simulink model "ce"  (R2016b)
settings: Solver=ode4  StartTime=0.0  StopTime=inf  FixedStep=0.001  RelTol=1e-3  EnableMultiTasking=on
undefined symbols (not defined in the file or in its folder): mdaadlink6208
libraries: dsparch4 x10
settings Model: SimulationMode=external  Creator=SHA  LastModifiedBy=Administrator
settings SolverCC: EnableConcurrentExecution=on
settings DataIOCC: SaveFormat=StructureWithTime
settings OptimizationCC: BlockReduction=off  OptimizeBlockIOStorage=off  BufferReuse=off  GlobalBufferReuse=off  ExpressionFolding=off  LocalBlockOutputs=off
settings HardwareCC: ProdBitPerPointer=32  ProdBitPerSizeT=32  ProdBitPerPtrDiffT=32  ProdLargestAtomicFloat=None  ProdWordSize=32  ProdLongLongMode=on  ProdHWDeviceType=Generic->32-bit x86 compatible
settings RTWCC: SystemTargetFile=slrt.tlc  TemplateMakefile=slrt_default_tmf  Description=Simulink Real-Time  RTWCompilerOptimization=on

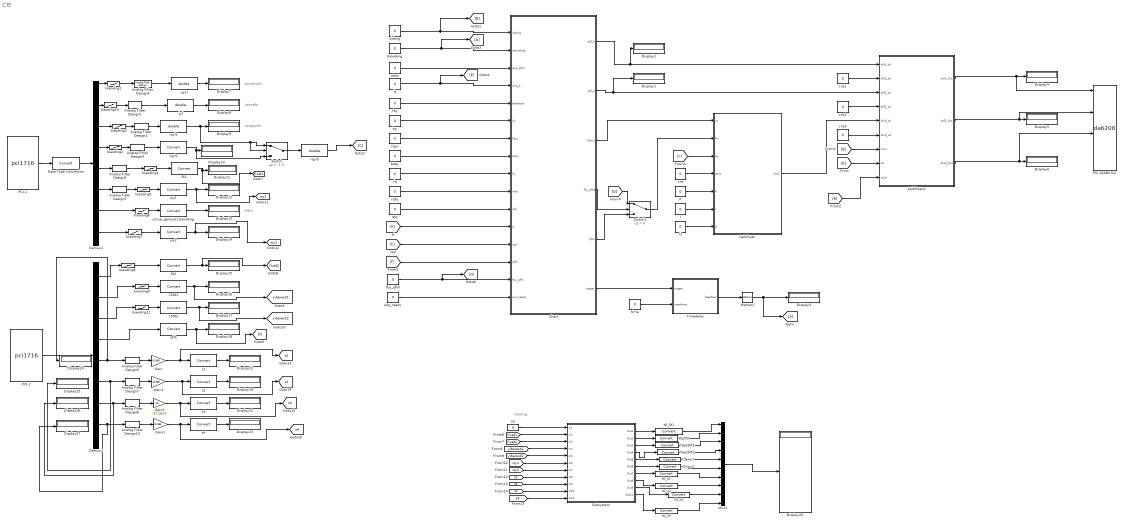
== system ce ==
  note: tiaoling
  note: qiyuanyali
  note: jianyafa
  note: rongqiyali
  note: weiyi
  150t1 : DataTypeConversion
  150t2 : DataTypeConversion
  5t1 : DataTypeConversion
  5t2 : DataTypeConversion
  Analog Filter Design{1..6} (6 alike) : dsparch4/Analog Filter Design  method=Butterworth  filttype=Lowpass  N=8  Wlo=2*pi*25  Whi=80  Rp=2  Rs=40
  Analog Filter Design{7..10} (4 alike) : dsparch4/Analog Filter Design  method=Butterworth  filttype=Lowpass  N=8  Wlo=2*pi*30  Whi=80  Rp=2  Rs=40
  Chart : Stateflow chart  TreatAsAtomicUnit=on
  D : Constant  Value=0
  Data Type Conversion : DataTypeConversion
  Demux1 : Demux  Outputs=16
  Demux2 : Demux  Outputs=16
  Display{1..27} (27 alike) : Display
  Gain : Gain  Gain=42.985
  Gain1 : Gain  Gain=42.985
  Gain2 : Gain  Gain=42.985
  Gain3 : Gain  Gain=-97.0874
  I : Constant  Value=0
  Memory : Memory
  Mux1 : Mux  Inputs=10
  P : Constant  Value=0
  PCI-1 : S-Function  FunctionName=pci1716  Parameters=[SampleTime SampleOffset], SLOT  SFunctionDeploymentMode=off  EnableBusSupport=off  mask(hitad3){Sample=0.001, SLOT=[2 13]}
      mask prompts: Sample "Sample Time:"
      mask help:
      | PCi1716
      | A/D Card
      | Developed by ZhaoJinsong
      | 2012.06.02
      mask init:
      | SampleTime = 0.001; SampleOffset=0;
      mask Help: helpview([docroot '/toolbox/xpc/pt_io_block_reference.html#xpcioref'])
      mask Display:
      | disp('PCI1716  ');
      | 
      | port_label('output',1 , 'OUT');
  PCI-2 : S-Function  FunctionName=pci1716  Parameters=[SampleTime SampleOffset], SLOT  SFunctionDeploymentMode=off  EnableBusSupport=off  mask(hitad3){Sample=0.001, SLOT=[2 12]}
      mask prompts: Sample "Sample Time:"
      mask help:
      | PCi1716
      | A/D Card
      | Developed by ZhaoJinsong
      | 2012.06.02
      mask init:
      | SampleTime = 0.001; SampleOffset=0;
      mask Help: helpview([docroot '/toolbox/xpc/pt_io_block_reference.html#xpcioref'])
      mask Display:
      | disp('PCI1716  ');
      | 
      | port_label('output',1 , 'OUT');
  "PCI-6208A DA " : S-Function  InitFcn=mdaadlink6208( 1 );  FunctionName=da6208  Parameters=channel, range, sampletime, pcislot, reset, initval  SFunctionDeploymentMode=off  EnableBusSupport=off  mask(da6208){channel=[1:8], range=4 to 20 ma, reset=[0], initval=[0], sampletime=0.001, pcislot=-1}
      mask prompts: channel "Channel vector:"; reset "Reset vector:"; initval "Initial value vector:"; sampletime "Sample time:"; pcislot "PCI slot (-1: autosearch):"
      mask help:
      | PCI-6208A
      | Adlink
      | Analog Output
      mask init:
      | [maskdisplay, reset, initval]= mdaadlink6208(2, channel, reset, initval, pcislot);
      | set_param(gcb,'MaskDisplay',maskdisplay);
      mask Help: helpview(fullfile(docroot, 'mapfiles', 'xpc.map'), 'Adlink_6208A_DA')
      mask TypeOptions range: 0 to 20 ma | 5 to 25 ma | 4 to 20 ma
      mask Display: disp('PCI-6208A\nAdlink\nAnalog Output');port_label('input',1,'1');port_label('input',2,'2');port_label('input',3,'3');port_label('input',4,'4');port_label('input',5,'5');port_label('input',6,'6');port_label('input',7,'7');port_label('input',8,'8');
  Subsystem : Subsystem
  Switch : Switch  Criteria=u2 > Threshold  Threshold=-1.5
  Switch1 : Switch  Criteria=u2 > Threshold
  Timedelay : Subsystem
  bdqy : Constant  Value=0
  biaoding{1..3,10} (4 alike) : Lookup  InputValues=[0 5]  Table=[0.01 2]  SaturateOnIntegerOverflow=on
  biaoding11 : Lookup  InputValues=[0 10]  Table=[0 150]  SaturateOnIntegerOverflow=on
  biaoding4 : Lookup  InputValues=[-0.16 10]  Table=[0 5]  SaturateOnIntegerOverflow=on
  biaoding5 : Lookup  InputValues=[-0.063 5]  Table=[0 100]  SaturateOnIntegerOverflow=on
  biaoding6 : Lookup  InputValues=[-0.052 5]  Table=[0 100]  SaturateOnIntegerOverflow=on
  biaoding7 : Lookup  InputValues=[-0.065 5]  Table=[0 100]  SaturateOnIntegerOverflow=on
  biaoding8 : Lookup  InputValues=[-0.002 10]  Table=[0 5]  SaturateOnIntegerOverflow=on
  biaoding9 : Lookup  InputValues=[0 10]  Table=[0 150]  SaturateOnIntegerOverflow=on
  by : Constant  Value=0
  cns{,1..3} (4 alike) : Constant  Value=0
  exp_ready : Constant  Value=0
  fby : Constant  Value=0
  fby_qfkk : Constant  Value=0
  fq : Constant  Value=0
  fqyc : Constant  Value=0
  jt : Constant  Value=0
  jyf : DataTypeConversion  OutDataTypeStr=double
  kaibihuan : Subsystem
  kaibihuan1 : Subsystem
  qffk : DataTypeConversion
  qfq : Constant  Value=0
  qyyl : DataTypeConversion  OutDataTypeStr=double
  rqfq : Constant  Value=0
  rqyl1 : DataTypeConversion  OutDataTypeStr=double
  rqyl2 : DataTypeConversion
  rqyl3 : DataTypeConversion  OutDataTypeStr=double
  s{1..4} (4 alike) : DataTypeConversion
  shoudong : Constant  Value=0
  start : Constant  Value=0
  t0 : Constant  Value=0
  t0_150t1 : DataTypeConversion
  t0_150t2 : DataTypeConversion
  t0_5t1 : DataTypeConversion
  t0_5t2 : DataTypeConversion
  t0_s{1..4} (4 alike) : DataTypeConversion
  t0_wy1 : DataTypeConversion
  t0_wy2 : DataTypeConversion
  time : Constant  Value=0
  wy1 : DataTypeConversion
  wy2 : DataTypeConversion
  yihuai_gensui11biandong : DataTypeConversion
  zidong : Constant  Value=0
  tag scope: fivet1=global, fivet2=global, s1=global, s2=global, s3=global, s4=global, wy1=global, wy2=global, yibaiwut1=global, yibaiwut2=global
  wires:
  start/1 -> Chart/3(exp_start)
  jt/1 -> [E], Chart/4(exp_jt)
  fby/1 -> Chart/5(feibaoya)
  by/1 -> Chart/6(by)
  fqyc/1 -> Chart/7(fqyc)
  Chart/3(kbhxz) -> kaibihuan/1(xz)
  Chart/2(dcf_2) -> kaibihuan1/3(dcf2_zd), Display1/1
  time/1 -> Timedelay/2(needtime)
  fq/1 -> Chart/9(fq)
  Chart/6(trigger) -> Timedelay/1(trigger)
  Timedelay/1(feedbool) -> Memory/1
  Memory/1 -> [A], Display3/1
  cns/1 -> kaibihuan/4(cons)
  P/1 -> kaibihuan/5(P)
  [A] -> Chart/12(sj)
  zidong/1 -> Chart/1(zidong), [B]
  I/1 -> kaibihuan/6(I)
  D/1 -> kaibihuan/7(D)
  [B] -> kaibihuan1/7(kzxz)
  cns1/1 -> kaibihuan1/2(dcf1_sd)
  cns2/1 -> kaibihuan1/4(dcf2_sd)
  cns3/1 -> kaibihuan1/6(dkqf_sd)
  kaibihuan/1(Out1) -> kaibihuan1/5(dkqf_zd)
  Chart/1(dcf_1) -> Display2/1, kaibihuan1/1(dcf1_zd)
  [C] -> Chart/13(rqyl)
  [C] -> kaibihuan/3(qy)
  qfq/1 -> Chart/11(qfq)
  rqfq/1 -> Chart/10(rqfq)
  kaibihuan1/1(dcf1_Out) -> "PCI-6208A DA "/1, Display4/1
  kaibihuan1/2(dcf2_Out) -> "PCI-6208A DA "/3, Display5/1
  kaibihuan1/3(dkqf_Out) -> "PCI-6208A DA "/5, Display6/1
  shoudong/1 -> Chart/2(shoudong), [D]
  Demux1/1 -> biaoding1/1
  Demux1/3 -> biaoding10/1
  Demux1/7 -> biaoding2/1
  PCI-1/1 -> Data Type Conversion/1
  Data Type Conversion/1 -> Demux1/1
  biaoding1/1 -> Analog Filter Design3/1
  biaoding3/1 -> Analog Filter Design2/1
  biaoding5/1 -> wy1/1
  biaoding10/1 -> Analog Filter Design1/1
  qyyl/1 -> Display7/1
  jyf/1 -> Display8/1
  rqyl2/1 -> Switch/3, Display10/1
  5t1/1 -> [fivet1], Display11/1
  wy1/1 -> [wy1], Display12/1
  biaoding6/1 -> yihuai_gensui11biandong/1
  yihuai_gensui11biandong/1 -> Display13/1
  biaoding7/1 -> wy2/1
  wy2/1 -> [wy2], Display14/1
  Demux1/15 -> biaoding7/1
  PCI-2/1 -> Demux2/1
  biaoding9/1 -> 150t1/1
  biaoding11/1 -> 150t2/1
  150t2/1 -> [yibaiwut2], Display17/1
  150t1/1 -> [yibaiwut1], Display16/1
  5t2/1 -> [fivet2], Display15/1
  Demux2/7 -> qffk/1
  qffk/1 -> [F], Display18/1
  [D] -> kaibihuan1/8(sd)
  [E] -> kaibihuan1/9(sd_jt)
  biaoding2/1 -> Analog Filter Design4/1
  Analog Filter Design2/1 -> rqyl1/1
  Analog Filter Design4/1 -> rqyl2/1
  Analog Filter Design1/1 -> jyf/1
  Analog Filter Design3/1 -> qyyl/1
  rqyl1/1 -> Switch/1, Switch/2, Display9/1
  bdqy/1 -> Chart/8(bdqy)
  Switch/1 -> rqyl3/1
  [F] -> Chart/14(qffk)
  fby_qfkk/1 -> [G], Chart/15(fby_qfkk)
  Chart/4(fby_qfsd) -> Switch1/2
  Chart/5(qfkk) -> Switch1/3
  Switch1/1 -> kaibihuan/2(kh)
  [G] -> Switch1/1
  exp_ready/1 -> Chart/16(exp_ready)
  rqyl3/1 -> [C]
  Mux1/1 -> Display20/1
  t0_5t1/1 -> Mux1/1
  t0_5t2/1 -> Mux1/2
  t0_150t1/1 -> Mux1/3
  t0_150t2/1 -> Mux1/4
  t0/1 -> Subsystem/1(In1)
  [fivet1] -> Subsystem/2(In2)
  [fivet2] -> Subsystem/3(In3)
  [yibaiwut1] -> Subsystem/4(In4)
  [yibaiwut2] -> Subsystem/5(In5)
  Subsystem/1(Out1) -> t0_5t1/1
  Subsystem/2(Out2) -> t0_5t2/1
  Subsystem/3(Out3) -> t0_150t1/1
  Subsystem/4(Out4) -> t0_150t2/1
  biaoding4/1 -> 5t1/1
  Demux2/1 -> biaoding8/1
  Demux1/9 -> Analog Filter Design6/1
  Demux1/5 -> biaoding3/1
  s1/1 -> Display22/1
  Gain/1 -> [s1], s1/1
  Demux2/9 -> Display24/1, Analog Filter Design9/1
  Demux2/3 -> biaoding9/1
  Demux2/5 -> biaoding11/1
  [wy1] -> Subsystem/6(In6)
  [wy2] -> Subsystem/7(In7)
  Subsystem/5(Out5) -> t0_wy1/1
  Subsystem/6(Out6) -> t0_wy2/1
  t0_wy1/1 -> Mux1/5
  t0_wy2/1 -> Mux1/6
  Demux1/11 -> Analog Filter Design5/1
  Demux1/13 -> biaoding6/1
  biaoding8/1 -> 5t2/1
  Analog Filter Design5/1 -> biaoding5/1
  Analog Filter Design6/1 -> biaoding4/1
  Gain2/1 -> [s2], s2/1
  Demux2/11 -> Display25/1, Analog Filter Design7/1
  Gain3/1 -> [s3], s3/1
  Gain1/1 -> [s4], s4/1
  Demux2/13 -> Display26/1, Analog Filter Design8/1
  Demux2/15 -> Display27/1, Analog Filter Design10/1
  s4/1 -> Display23/1
  s3/1 -> Display21/1
  s2/1 -> Display19/1
  [s1] -> Subsystem/8(In8)
  [s2] -> Subsystem/9(In9)
  [s3] -> Subsystem/10(In10)
  [s4] -> Subsystem/11(In11)
  t0_s1/1 -> Mux1/7
  t0_s2/1 -> Mux1/8
  t0_s3/1 -> Mux1/9
  t0_s4/1 -> Mux1/10
  Subsystem/7(Out7) -> t0_s1/1
  Subsystem/8(Out8) -> t0_s2/1
  Subsystem/9(Out9) -> t0_s3/1
  Subsystem/10(Out10) -> t0_s4/1
  Analog Filter Design7/1 -> Gain2/1
  Analog Filter Design8/1 -> Gain3/1
  Analog Filter Design9/1 -> Gain/1
  Analog Filter Design10/1 -> Gain1/1

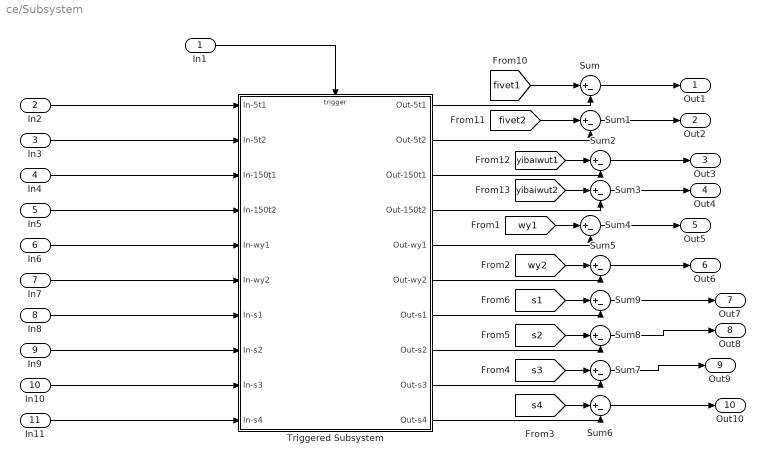
== system ce/Subsystem ==
  In1 : Inport
  In2 : Inport  Port=2
  In3 : Inport  Port=3
  In4 : Inport  Port=4
  In5 : Inport  Port=5
  In6 : Inport  Port=6
  In7 : Inport  Port=7
  In8 : Inport  Port=8
  In9 : Inport  Port=9
  In10 : Inport  Port=10
  In11 : Inport  Port=11
  Sum{,1..9} (10 alike) : Sum  Inputs=|+-
  Triggered Subsystem : Subsystem  TreatAsAtomicUnit=on
  Out1 : Outport
  Out2 : Outport  Port=2
  Out3 : Outport  Port=3
  Out4 : Outport  Port=4
  Out5 : Outport  Port=5
  Out6 : Outport  Port=6
  Out7 : Outport  Port=7
  Out8 : Outport  Port=8
  Out9 : Outport  Port=9
  Out10 : Outport  Port=10
  wires:
  In2/1 -> Triggered Subsystem/1(In-5t1)
  In4/1 -> Triggered Subsystem/3(In-150t1)
  [fivet2] -> Sum1/1
  In3/1 -> Triggered Subsystem/2(In-5t2)
  Triggered Subsystem/3(Out-150t1) -> Sum2/2
  [fivet1] -> Sum/1
  Sum/1 -> Out1/1
  Sum1/1 -> Out2/1
  Sum3/1 -> Out4/1
  Sum2/1 -> Out3/1
  [yibaiwut2] -> Sum3/1
  [yibaiwut1] -> Sum2/1
  Triggered Subsystem/2(Out-5t2) -> Sum1/2
  In5/1 -> Triggered Subsystem/4(In-150t2)
  Triggered Subsystem/1(Out-5t1) -> Sum/2
  In1/1 -> Triggered Subsystem/Trigger
  Triggered Subsystem/4(Out-150t2) -> Sum3/2
  Sum4/1 -> Out5/1
  [wy1] -> Sum4/1
  Triggered Subsystem/5(Out-wy1) -> Sum4/2
  Sum5/1 -> Out6/1
  [wy2] -> Sum5/1
  Triggered Subsystem/6(Out-wy2) -> Sum5/2
  In6/1 -> Triggered Subsystem/5(In-wy1)
  In7/1 -> Triggered Subsystem/6(In-wy2)
  In11/1 -> Triggered Subsystem/10(In-s4)
  In10/1 -> Triggered Subsystem/9(In-s3)
  In9/1 -> Triggered Subsystem/8(In-s2)
  In8/1 -> Triggered Subsystem/7(In-s1)
  Sum6/1 -> Out10/1
  [s4] -> Sum6/1
  Triggered Subsystem/10(Out-s4) -> Sum6/2
  Sum7/1 -> Out9/1
  [s3] -> Sum7/1
  Triggered Subsystem/9(Out-s3) -> Sum7/2
  Sum8/1 -> Out8/1
  [s2] -> Sum8/1
  Triggered Subsystem/8(Out-s2) -> Sum8/2
  Sum9/1 -> Out7/1
  [s1] -> Sum9/1
  Triggered Subsystem/7(Out-s1) -> Sum9/2

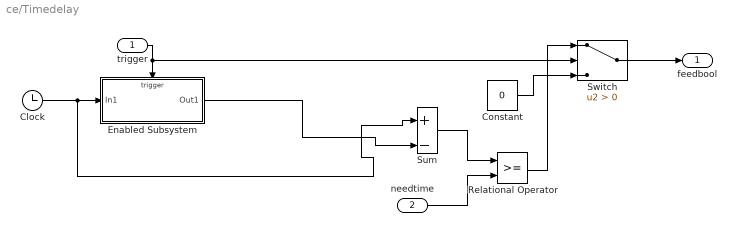
== system ce/Timedelay ==
  trigger : Inport
  needtime : Inport  Port=2
  Clock : Clock
  Constant : Constant  Value=0
  Enabled Subsystem : Subsystem  TreatAsAtomicUnit=on
  Relational Operator : RelationalOperator  OutDataTypeStr=boolean  RndMeth=Simplest
  Sum : Sum  Inputs=|+-
  Switch : Switch  Criteria=u2 > Threshold
  feedbool : Outport
  wires:
  Clock/1 -> Sum/1, Enabled Subsystem/1(In1)
  Enabled Subsystem/1(Out1) -> Sum/2
  Sum/1 -> Relational Operator/1
  needtime/1 -> Relational Operator/2
  trigger/1 -> Switch/2, Enabled Subsystem/Trigger
  Relational Operator/1 -> Switch/1
  Constant/1 -> Switch/3
  Switch/1 -> feedbool/1

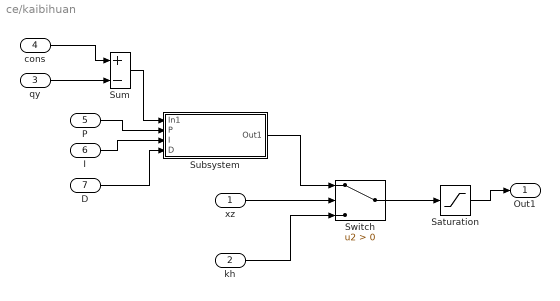
== system ce/kaibihuan ==
  xz : Inport
  kh : Inport  Port=2
  qy : Inport  Port=3
  cons : Inport  Port=4
  P : Inport  Port=5
  I : Inport  Port=6
  D : Inport  Port=7
  Saturation : Saturate  UpperLimit=5  LowerLimit=0
  Subsystem : Subsystem
  Sum : Sum  Inputs=|+-
  Switch : Switch  Criteria=u2 > Threshold
  Out1 : Outport
  wires:
  xz/1 -> Switch/2
  cons/1 -> Sum/1
  qy/1 -> Sum/2
  Sum/1 -> Subsystem/1(In1)
  P/1 -> Subsystem/2(P)
  I/1 -> Subsystem/3(I)
  D/1 -> Subsystem/4(D)
  Subsystem/1(Out1) -> Switch/1
  kh/1 -> Switch/3
  Saturation/1 -> Out1/1
  Switch/1 -> Saturation/1

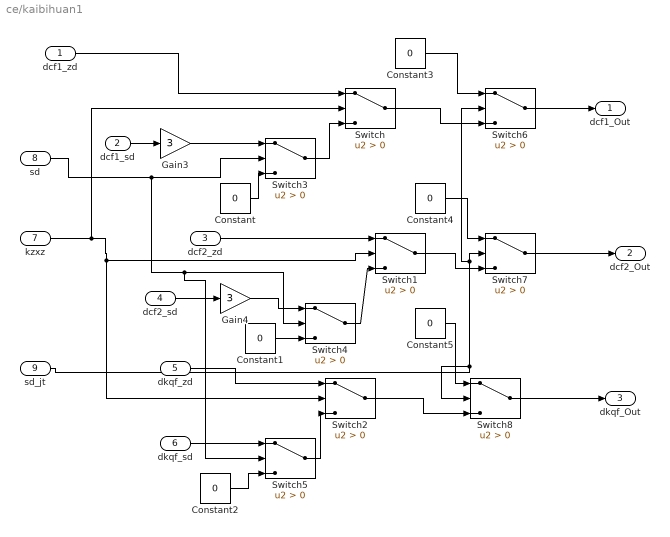
== system ce/kaibihuan1 ==
  dcf1_zd : Inport
  dcf1_sd : Inport  Port=2
  dcf2_zd : Inport  Port=3
  dcf2_sd : Inport  Port=4
  dkqf_zd : Inport  Port=5
  dkqf_sd : Inport  Port=6
  kzxz : Inport  Port=7
  sd : Inport  Port=8
  sd_jt : Inport  Port=9
  Constant{,1..5} (6 alike) : Constant  Value=0
  Gain3 : Gain  Gain=3
  Gain4 : Gain  Gain=3
  Switch{,1..8} (9 alike) : Switch  Criteria=u2 > Threshold
  dcf1_Out : Outport
  dcf2_Out : Outport  Port=2
  dkqf_Out : Outport  Port=3
  wires:
  dcf1_zd/1 -> Switch/1
  dcf2_zd/1 -> Switch1/1
  dkqf_zd/1 -> Switch2/1
  dcf1_sd/1 -> Gain3/1
  dcf2_sd/1 -> Gain4/1
  kzxz/1 -> Switch/2, Switch2/2, Switch1/2
  Switch3/1 -> Switch/3
  Gain3/1 -> Switch3/1
  Constant/1 -> Switch3/3
  Gain4/1 -> Switch4/1
  Constant1/1 -> Switch4/3
  Switch4/1 -> Switch1/3
  Switch5/1 -> Switch2/3
  dkqf_sd/1 -> Switch5/1
  sd/1 -> Switch5/2, Switch4/2, Switch3/2
  Constant2/1 -> Switch5/3
  Switch6/1 -> dcf1_Out/1
  Switch7/1 -> dcf2_Out/1
  Switch2/1 -> Switch8/3
  Switch8/1 -> dkqf_Out/1
  Switch1/1 -> Switch7/3
  Switch/1 -> Switch6/3
  Constant3/1 -> Switch6/1
  Constant4/1 -> Switch7/1
  Constant5/1 -> Switch8/1
  sd_jt/1 -> Switch8/2, Switch6/2, Switch7/2

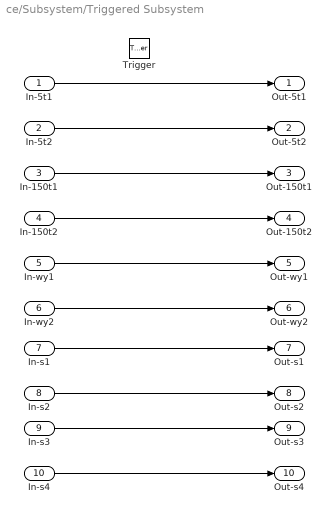
== system ce/Subsystem/Triggered Subsystem ==
  In-5t1 : Inport
  In-5t2 : Inport  Port=2
  In-150t1 : Inport  Port=3
  In-150t2 : Inport  Port=4
  In-wy1 : Inport  Port=5
  In-wy2 : Inport  Port=6
  In-s1 : Inport  Port=7
  In-s2 : Inport  Port=8
  In-s3 : Inport  Port=9
  In-s4 : Inport  Port=10
  Trigger : TriggerPort  VariantControl=Variant
  Out-5t1 : Outport
  Out-5t2 : Outport  Port=2
  Out-150t1 : Outport  Port=3
  Out-150t2 : Outport  Port=4
  Out-wy1 : Outport  Port=5
  Out-wy2 : Outport  Port=6
  Out-s1 : Outport  Port=7
  Out-s2 : Outport  Port=8
  Out-s3 : Outport  Port=9
  Out-s4 : Outport  Port=10
  wires:
  In-5t1/1 -> Out-5t1/1
  In-5t2/1 -> Out-5t2/1
  In-150t1/1 -> Out-150t1/1
  In-150t2/1 -> Out-150t2/1
  In-wy1/1 -> Out-wy1/1
  In-wy2/1 -> Out-wy2/1
  In-s1/1 -> Out-s1/1
  In-s2/1 -> Out-s2/1
  In-s3/1 -> Out-s3/1
  In-s4/1 -> Out-s4/1

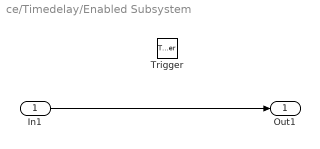
== system ce/Timedelay/Enabled Subsystem ==
  In1 : Inport
  Trigger : TriggerPort  VariantControl=Variant  PortDimensions=1
  Out1 : Outport
  wires:
  In1/1 -> Out1/1

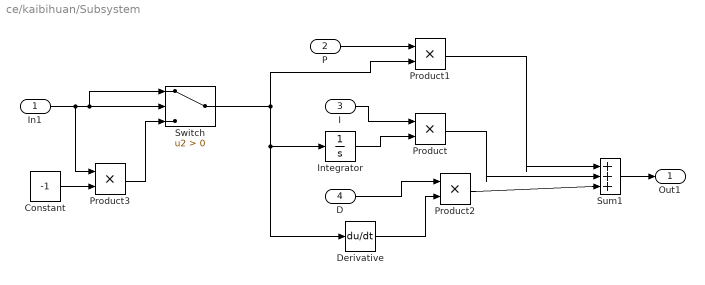
== system ce/kaibihuan/Subsystem ==
  In1 : Inport
  P : Inport  Port=2
  I : Inport  Port=3
  D : Inport  Port=4
  Constant : Constant  Value=-1
  Derivative : Derivative
  Integrator : Integrator
  Product{,1..3} (4 alike) : Product
  Sum1 : Sum  Inputs=|+++
  Switch : Switch  Criteria=u2 > Threshold
  Out1 : Outport
  wires:
  Integrator/1 -> Product/2
  I/1 -> Product/1
  P/1 -> Product1/1
  D/1 -> Product2/1
  Derivative/1 -> Product2/2
  Product1/1 -> Sum1/1
  Product/1 -> Sum1/2
  Product2/1 -> Sum1/3
  Sum1/1 -> Out1/1
  In1/1 -> Product3/1, Switch/1, Switch/2
  Constant/1 -> Product3/2
  Product3/1 -> Switch/3
  Switch/1 -> Derivative/1, Integrator/1, Product1/2

== stateflow chart ce/Chart ==
  state kong
  state fby
    state fby_action2
      en:
      dcf_1 =5;
      dcf_2 =0;
    state fby_action3
      en:
      dcf_2 =5;
      dcf_1 =0;
    state fby_action1
      en:
      fby_qfsd=1;
    (default) -> fby_action1
    fby_action2 -> fby_action3 : [rqyl>=bdqy]
    fby_action1 -> fby_action2 : [qffk>=(fby_qfkk-0.2)&&exp_start==1]
  state exp_fq
    state exp_rqfq
      en:
      dcf_1=0;
      dcf_2 =5;
      kbhxz =0;
      qfkk =0;
    state kong1
      en:
      fby_qfsd=0;
    state exp_qfq
      en:
      dcf_1=5;
      dcf_2 =5;
      kbhxz =0;
      qfkk =5;
    (default) -> kong1
    kong1 -> exp_rqfq [order 1] : [rqfq==1&&qfq==0]
    kong1 -> exp_qfq [order 2] : [rqfq==0&&qfq==1]
    exp_rqfq -> exp_qfq : [qfq==1]
    exp_qfq -> exp_rqfq : [rqfq==1]
  state exp_ready
    en:
    dcf_1=0;
    dcf_2 =0;
    trigger =0;
    kbhxz =0;
    qfkk =0;
    fby_qfsd=0;
  note: baoya
  state by
    state bysjgd_action1
      en:
      dcf_1 =5;
      kbhxz =1;
      dcf_2 =0;
    state bysjgd_action3
      en:
      dcf_2 =5;
      kbhxz =0;
      qfkk =0;
      dcf_1 =0;
    state bysjgd_action2
      en:
      dcf_1 =0;
      dcf_2 =0;
      trigger =1;
    (default) -> bysjgd_action1
    bysjgd_action1 -> bysjgd_action3 [order 1] : [sj ==1]
    bysjgd_action1 -> bysjgd_action2 [order 2] : [rqyl>bdqy]
    bysjgd_action2 -> bysjgd_action1 [order 1] : [rqyl<bdqy]
    bysjgd_action2 -> bysjgd_action3 [order 2] : [sj ==1]
  note: fangqiyanchi
  state fqyc
    state fqyc_action2
      en:
      dcf_1 =5;
      dcf_2 =0;
    state fqyc_action3
      en:
      trigger =1;
      dcf_1 =0;
    state fqyc_action4
      en:
      dcf_1 =0;
      dcf_2 =5;
    state fqyc_action1
      en:
      fby_qfsd=1;
    (default) -> fqyc_action1
    fqyc_action3 -> fqyc_action4 : [sj ==1]
    fqyc_action2 -> fqyc_action3 : [rqyl>=bdqy]
    fqyc_action1 -> fqyc_action2 : [qffk>=(fby_qfkk-0.2)&&exp_start==1]
  (default) -> kong
  kong -> (junction 199) : [zidong==1&&shoudong==0]
  exp_ready -> kong [order 3] : [zidong==0&&shoudong==1]
  fby -> exp_ready : [(exp_start==0&&exp_ready==0)||exp_jt ==1]
  (junction 6) -> fby [order 1] : [feibaoya==1&&rqyl<bdqy&&exp_ready==1]
  (junction 199) -> exp_fq [order 1] : [fq==1]
  (junction 199) -> exp_ready [order 2] : [fq==0]
  exp_ready -> (junction 6) [order 1] : [exp_jt ==0]
  (junction 6) -> by [order 2] : [by==1&&rqyl<bdqy&&exp_start==1]
  (junction 6) -> fqyc [order 3] : [fqyc==1&&rqyl<bdqy&&exp_ready==1]
  exp_fq -> exp_ready : [fq==0||exp_jt ==1]
  exp_ready -> exp_fq [order 2] : [fq==1]
  by -> exp_ready : [exp_start==0||exp_jt ==1]
  fqyc -> exp_ready : [(exp_start==0&&exp_ready==0)||exp_jt ==1]
  data: zidong input double; shoudong input double; exp_start input double; exp_jt input double; feibaoya input double; by input double; fqyc input double; bdqy input double; dcf_1 output double; dcf_2 output double; kbhxz output double; fby_qfsd output; qfkk output double; trigger output double; fq input double; rqfq input double; qfq input double; sj input double; rqyl input double; qffk input double; fby_qfkk input; exp_ready input
